simulink model "TruckBenchmark"  (R2023a)
settings: Solver=FixedStepAuto  StartTime=0.0  StopTime=sim_time  FixedStep=control.Ts  MaxStep=1  RelTol=1e-3  EnableMultiTasking=on
StartFcn:
  | tic
StopFcn:
  | simt=toc;
  | fprintf('Simulation time %.3f s\n',simt)
  | TruckBenchmark_Evaluation
values from neighbouring files (symbols this model uses):
  attack_duration = input('Enter the duration of each attack: ')    [RunMe.m]
  attack_freq = input('Enter the desired frequency of attack: ')    [RunMe.m]
  attack_time = input('Enter the time for attack: ')    [RunMe.m]
  attack_type = input('Select the type of Attack (1= Fuzzy, 2=spoofing, 3=Plateau, 4=Replay Attack, 5 = GAttack, 6= C-GAttack, 7= No Attack, 8 = Denial of Service):')    [RunMe.m]
  can_sample_time = 0.001    [runSim.m]
  clutch_pos = TruckBenchmark_Result.find('clutch_pos').Values    [TruckBenchmark_Evaluation.m]
  control =     [TruckBenchmark_Control.mat]
  cruise_profile = input('Select Cruise Profile (Step decrease = 1, Constant 80kph = 2): ')    [RunMe.m]
  curr_gear = TruckBenchmark_Result.find('curr_gear').Values    [TruckBenchmark_Evaluation.m]
  DoS = 0    [RunMe.m]
  gattack_data = interp1(original_time, data, desired_time, 'linear')    [RunMe.m]
  gattack_time = desired_time    [RunMe.m]
  k_slope = TruckBenchmark_Result.find('k_slope').Values    [TruckBenchmark_Evaluation.m]
  lambda = TruckBenchmark_Result.find('lambda').Values    [TruckBenchmark_Evaluation.m]
  model =     [TruckBenchmark_Data.mat]
  n_engine = TruckBenchmark_Result.find('n_engine').Values    [TruckBenchmark_Evaluation.m]
  road = scenario.road    [runSim.m]
  scenario =     [Sodertalje_Norrkoping_Scenario.mat]
  sim_time = input('Enter the total simulation time: ')    [RunMe.m]
  spoofed_value = input('Set the spoofing value:')    [RunMe.m]
  ts = struct('orig_30kph', ts_orig_30kph, 'gen_30kph', ts_gen_30kph, 'orig_40kph', ts_orig_40kph, 'gen_40kph', ts_gen_40kph, 'orig_50kph', ts_orig_50kph, 'gen_50kph', ts_gen_50kph, 'orig_60kph', ts_orig_60kph, 'gen_60kph', ts_gen_60kph,'orig_70kph', ts_orig_70kph, 'gen_70kph', ts_gen_70kph, 'orig_80kph', ts_orig_80kph, 'gen_80kph', ts_gen_80kph, 'orig_90kph', ts_orig_90kph, 'gen_90kph', ts_gen_90kph)    [data_to_mat.m]
  v_vehicle = 0    [RunMe.m]    (also in TruckBenchmark_Evaluation.m = TruckBenchmark_Result.find('v_vehicle').Values)
undefined symbols (not defined in the file or in its folder): canChannel, CCVS, DiscIntNeverNeededParam, dm_airInlet, EGF1, ESSI, ETC2, gcbh, IMT1, n_t, p_inletManifold, r_egr, VD, VDHR, x_distance
libraries: j1939protocollib x25, simulink x5, canlib x2, j1939tllib x2, canmsglib x1, vntj1939tllib x1, slpidlib x1
(part 4 of 4)

== system TruckBenchmark/Vehicle Model/ICE/Turbo/Turbine/eta_tm ==
  omega_t : Inport
  T_em : Inport  Port=2
  PI_t : Inport  Port=3
  BSR : Fcn  Expr=R_t*u[1]/sqrt(2*c_pe*u[2]*(1-u[3]^(1-1/gamma_e)))
  Fcn eta_t : Fcn  Expr=eta_tmmax-u[1]*(u[2]-BSR_opt)^2
  Mux1 : Mux  Inputs=2
  Mux4 : Mux  Inputs=3
  Saturation : Saturate  UpperLimit=2*BSR_opt  LowerLimit=0
  Saturation1 : Saturate  UpperLimit=1  LowerLimit=0.2
  c_m : Subsystem
  eta_tm : Outport  VectorParamsAs1DForOutWhenUnconnected=off
  tag scope: BSR=global
  wires:
  c_m/1(c_m) -> Mux1/1
  Saturation/1 -> [BSR], Mux1/2
  Mux1/1 -> Fcn eta_t/1
  Saturation1/1 -> eta_tm/1
  Fcn eta_t/1 -> Saturation1/1
  PI_t/1 -> Mux4/3
  T_em/1 -> Mux4/2
  omega_t/1 -> c_m/1(omega_t), Mux4/1
  BSR/1 -> Saturation/1
  Mux4/1 -> BSR/1

== system TruckBenchmark/Vehicle Model/ICE/Turbo/Compressor/DeltaT_c/eta_c ==
  W_c : Inport
  PI_c : Inport  Port=2
  Constant2 : Constant  Value=0.2
  Fcn eta_c : Fcn  Expr=eta_cmax-u
  Matrix Gain : Gain  Gain=Q_c  Multiplication=Matrix(K*u)  SaturateOnIntegerOverflow=on  OutDataTypeStr=Inherit: Same as input  ParamDataTypeStr=Inherit: Same as input
  MinMax2 : MinMax  Function=max  Inputs=2  InputSameDT=on  SaturateOnIntegerOverflow=on
  Mux6 : Mux  Inputs=2
  Product : Product  Multiplication=Matrix(*)  SaturateOnIntegerOverflow=on  OutDataTypeStr=Inherit: Same as first input
  chi1 : Fcn  Expr=u-w_copt
  chi2 : Fcn  Expr=u-pi_copt
  pi_c : Fcn  Expr=(u-1)^c_pi
  transp : Math  Operator=transpose  SignedPower=on
  eta_c : Outport  VectorParamsAs1DForOutWhenUnconnected=off
  wires:
  W_c/1 -> chi1/1
  MinMax2/1 -> eta_c/1
  PI_c/1 -> pi_c/1
  Constant2/1 -> MinMax2/2
  Fcn eta_c/1 -> MinMax2/1
  Product/1 -> Fcn eta_c/1
  Matrix Gain/1 -> Product/2
  transp/1 -> Product/1
  Mux6/1 -> transp/1, Matrix Gain/1
  chi2/1 -> Mux6/2
  chi1/1 -> Mux6/1
  pi_c/1 -> chi2/1

== system TruckBenchmark/Vehicle Model/ICE/Turbo/Compressor/Sub W_c/PHI_c ==
  PI_c : Inport
  T_bc : Inport  Port=2
  omega_t : Inport  Port=3
  Constant : Constant  Value=0
  Constant1 : Constant  Value=0
  Constant2 : Constant  Value=0
  Constant3 : Constant  Value=0.1
  MinMax{,1..3} (4 alike) : MinMax  Function=max  Inputs=2  InputSameDT=on  SaturateOnIntegerOverflow=on
  Mux1 : Mux  Inputs=2
  Mux2 : Mux  Inputs=2
  Mux5 : Mux  Inputs=3
  PSI_c : Fcn  Expr=2*c_pa*u[2]*(u[1]^(1-1/gamma_a)-1)/(R_c^2*u[3]^2)
  c_phi1 : Polyval  Coefs=c_wphiVec
  c_psi1 : Polyval  Coefs=c_wpsiVec
  fcn : Fcn  Expr=1-u[2]*(u[1]-c_psi2)^2
  fcn1 : Fcn  Expr=c_phi2+sqrt(u[1]/u[2])
  PHI_c : Outport  VectorParamsAs1DForOutWhenUnconnected=off
  wires:
  Constant3/1 -> MinMax3/2
  MinMax3/1 -> Mux2/2
  c_phi1/1 -> MinMax3/1
  MinMax2/1 -> PHI_c/1
  fcn1/1 -> MinMax2/2
  Constant2/1 -> MinMax2/1
  Mux2/1 -> fcn1/1
  MinMax/1 -> Mux2/1
  fcn/1 -> MinMax/2
  Constant/1 -> MinMax/1
  MinMax1/1 -> Mux1/2
  c_psi1/1 -> MinMax1/1
  Constant1/1 -> MinMax1/2
  Mux1/1 -> fcn/1
  PSI_c/1 -> Mux1/1
  omega_t/1 -> c_phi1/1, c_psi1/1, Mux5/3
  T_bc/1 -> Mux5/2
  PI_c/1 -> Mux5/1
  Mux5/1 -> PSI_c/1

== system TruckBenchmark/Vehicle Model/ICE/Turbo/Turbine/Sub W_t/f_vgt ==
  u_vgt : Inport
  Constant : Constant  Value=0
  Constant1 : Constant  Value=0
  Fcn f_vgt : Fcn  Expr=c_f2+c_f1*sqrt(u)
  Fcn1 : Fcn  Expr=1-((u-c_vgt2)/c_vgt1)^2
  MinMax : MinMax  Function=max  Inputs=2  InputSameDT=on  SaturateOnIntegerOverflow=on
  MinMax1 : MinMax  Function=max  Inputs=2  InputSameDT=on  SaturateOnIntegerOverflow=on
  f_vgt : Outport  VectorParamsAs1DForOutWhenUnconnected=off
  wires:
  MinMax1/1 -> f_vgt/1
  Fcn f_vgt/1 -> MinMax1/1
  Constant1/1 -> MinMax1/2
  MinMax/1 -> Fcn f_vgt/1
  Constant/1 -> MinMax/2
  Fcn1/1 -> MinMax/1
  u_vgt/1 -> Fcn1/1

== system TruckBenchmark/Vehicle Model/ICE/Turbo/Turbine/eta_tm/c_m ==
  omega_t : Inport
  Constant : Constant  Value=c_mVec(2)
  MinMax : MinMax  Function=max  Inputs=2  InputSameDT=on  SaturateOnIntegerOverflow=on
  Switch PSI : Switch  Threshold=w_tlin  InputSameDT=off
  c_m linear : Fcn  Expr=c_mlin*(u-c_mVec(2))/(w_tlin-c_mVec(2))
  c_m power : Fcn  Expr=c_mVec(1)*(u-c_mVec(2))^c_mVec(3)
  c_m : Outport  VectorParamsAs1DForOutWhenUnconnected=off
  wires:
  Switch PSI/1 -> c_m/1
  c_m linear/1 -> Switch PSI/3
  c_m power/1 -> Switch PSI/1
  omega_t/1 -> MinMax/2
  Constant/1 -> MinMax/1
  MinMax/1 -> c_m linear/1, Switch PSI/2, c_m power/1

== matlab function TruckBenchmark/Controller/Controller/cruise_set ==
  data: time input; cruise_set_speed output
function cruise_set_speed = switch_sig(time)
    % Define time constraint parameters
    %switch_time = 150; % Time to switch signals (in seconds)
    to = 100;
    % Initialize mux input
    cruise_set_speed = zeros(size(time));
    
    % Select signal 1 for the first part of the time vector
    if (time <= to )
        cruise_set_speed = 90;
    elseif (time > to && time<=to+50) 
        cruise_set_speed = 90;
    elseif (time > to+50 && time<=to+150) 
        cruise_set_speed = 80;
    elseif (time > to+150 && time<=to+250) 
        cruise_set_speed = 70;
    elseif (time > to+250 && time<=to+350) 
        cruise_set_speed = 60;
    elseif (time > to+350 && time<=to+450) 
        cruise_set_speed = 50;
    elseif (time > to+450 && time<=to+550) 
        cruise_set_speed = 40;
        %cruise_set_speed = 50;
    elseif (time > to+550) 
        cruise_set_speed = 30;
        %cruise_set_speed = 50;




    
    
end

== matlab function TruckBenchmark/Controller/CAN TX//RX/Attack_select ==
  data: GAttack input; output output; CGAttack input
function output = switch_sig(GAttack, CGAttack)
    % Define time constraint parameters
    switch_signal = attack_type; % Time to apply attack (no attack if at sim stop time)
    %switch_time = max(simTime); % Time to apply attack (Gattack)
    %switch_time = max(simTime); % Time to apply attack (CGattack)

    % Initialize mux input
    output = zeros(size(GAttack));
    
    % Select signal 1 for the first part of the time vector
    if (switch_signal == 1)
        output = GAttack;
    elseif (switch_signal == 2) 
        output = CGAttack;
    else
        output = 0;
    
    
end

== matlab function TruckBenchmark/Controller/CAN TX//RX/Attack Block/Attack_Block2 ==
  data: time input; mux_input output; attack_time input; attack_freq input; attack_duration input; sim_time input
function mux_input = switch_sig(time, attack_time, attack_freq, attack_duration, sim_time)
    % Initialize mux input as a vector of zeros with the same size as time
    mux_input = zeros(size(time));

    % Define the period between consecutive attacks
    attack_interval = (sim_time - attack_time) / (attack_freq);

    % Iterate through each time step
    for i = 1:length(time)
        % For each attack, determine if the time is within the attack period
        for j = 0:attack_freq-1
            current_attack_start = attack_time + j * attack_interval;
            current_attack_end = current_attack_start + attack_duration;
            
            % Check if the current time falls within the attack period
            if time(i) >= current_attack_start && time(i) <= current_attack_end
                mux_input(i) = 1;  % Set the signal to 1 during the attack
            end
        end
    end
end

== matlab function TruckBenchmark/Controller/Controller/P speed control ==
  data: v_ref input; v_speed input; u output; p_im input; curr_gear input; gear input; v_err output
function [u, v_err] = P(v_ref,v_speed,p_im,curr_gear,gear)
%#codegen


Kp      = 300;
v_err   = v_ref - v_speed;
u       = v_err * Kp;

% smoke limiter
K_smoke = 0.0012;
u_max=K_smoke*p_im;

% handle upshifts where the speed changes rapidly and the slowly sampled
% controller lags behind.
persistent last_gear second_last_gear

if isempty(last_gear)
  last_gear=4;
  second_last_gear=4;
end
if second_last_gear<curr_gear,
  u_max=u_max*.7;
end

second_last_gear=last_gear;
last_gear=curr_gear;
u=min(u,u_max);

== matlab function TruckBenchmark/Vehicle Model/Transmission Control Unit ==
  settings: updateMethod=DISCRETE
  data: gear_ref input; clutch output; gear_out output; time input
function [clutch,gear_out]  = TCU(gear_ref,time)
%#codegen
% Transmission control unit
persistent previous_gear incoming_gear last_state
persistent state t_start last_call
t_declutch=0.5;
t_speed_sync=1.0;
t_onclutch=0.5;


% run initialization
if isempty(state)
  % Initial state
  state=0;
  % Need to set varibles (some to dummy) so that codegen gets to know the size of the
  % persistent variables
  previous_gear=4;
  incoming_gear=4;
  t_start=0;
  previous_gear=gear_ref;
  last_call=time;
  last_state=state;
end
  
% Check if Simulink is restarting with smaller step reduction
if time < last_call,
  if state > 0,
    % disp(['Time reversed during gearchange']);
    if time - t_start < t_declutch,
      state=1;
    elseif time - t_start < t_declutch+t_speed_sync,
      state=2;
    elseif time - t_start < t_declutch+t_speed_sync+t_onclutch
      % backing state_machine
      state=3;
    else
      state=0;
    end
  end
end

last_call=time;
last_state=state;

% Run the state machine
switch state,
  case 0, % 'normal'
    if (gear_ref~=previous_gear)
      t_start=time;
      incoming_gear=gear_ref;
      state=1;
    end
    clutch=1;
    gear_out=previous_gear;
  case 1, % 'ramp_down',
    if ((time-t_start)>t_declutch)
      state=2;
      clutch=0;
    else
      clutch=1-(time-t_start)/t_declutch;
    end    
    gear_out=previous_gear;
  case 2, % 'change_gear',
    if (time>(t_start+t_declutch+t_speed_sync))
      state=3; % 'ramp_up';
      clutch=(time-(t_start+t_declutch+t_speed_sync))/t_onclutch;
    else
      clutch=0;
    end
    gear_out=incoming_gear;
  case 3, % 'ramp_up',
    if (time>(t_start+t_declutch+t_speed_sync+t_onclutch))
      state=0; %'normal';
      clutch=1;
    else
      clutch=(time-(t_start+t_declutch+t_speed_sync))/t_onclutch;
    end
    gear_out=incoming_gear;
    previous_gear=incoming_gear;
  otherwise
    error('Unknown state');
end

== matlab function TruckBenchmark/Vehicle Model/Fuel consumption dm^3//(100km) ==
  data: m_fuelTot input; x_distance input; fuelConsumption output
function fuelConsumption = fcn(m_fuelTot,x_distance)
%#codegen
rho_fuel = 0.8;                               % kg/m^2
if x_distance > 1000
    fuelConsumption = m_fuelTot / (rho_fuel * x_distance / 100000 );   % dm^3/(100km)
else
    fuelConsumption = nan;
end

== matlab function TruckBenchmark/Controller/Controller/PI speed control1 ==
  data: k_slopeVector input; k_slope output; x_distanceVector input; currentPos input
function k_slope = slope(k_slopeVector ,  x_distanceVector, currentPos)
%#codegen

% This function is not implemented.
k_slope      = 0;

== matlab function TruckBenchmark/Controller/Controller/Gear control ==
  data: n_ice input; gear_ref output; curr_gear input; clutch input
function gear_ref  = gearbox_control(n_ice, curr_gear, clutch)
%#codegen

% Define persistant variables
persistent curr_gear_ref

% initialize persistant variable
if isempty(curr_gear_ref)
    curr_gear_ref=4;
end

n_gearUpshift = 1250;
n_gearDoubleUpshift = 1800;
n_gearDownshift = 900;
gearMax   = 14;
gearMin   = 4;

if curr_gear_ref~=curr_gear || clutch~=1; %Gear in progress - keep current gear reference
    gear_ref = curr_gear_ref;     
elseif n_ice > n_gearUpshift && curr_gear < gearMax %Shift upp  
    if n_ice > n_gearDoubleUpshift && curr_gear < gearMax-1 %Shift up two gears
        gear_ref = curr_gear + 2;
    else % Shift up one gear
        gear_ref = curr_gear + 1;
    end 
elseif n_ice < n_gearDownshift && curr_gear > gearMin %Shift down
    gear_ref = curr_gear - 1;
else %No shift - keep current gear
    gear_ref = curr_gear;
end

gear_ref = min(max(gear_ref,gearMin),gearMax); %Should not be necissairy

curr_gear_ref=gear_ref;

== matlab function TruckBenchmark/Controller/Controller/PI speed control ==
  data: v_ref input; v_speed input; u output; p_im input; curr_gear input; gear input; v_err output; u_int input; u_diff input
function [u, v_err] = PI(v_ref,v_speed,p_im,curr_gear,gear, u_int, u_diff)
%#codegen
persistent last_v_err last_t

Kp      = 400;
Ki      = 0.05; % Increase the integration gain
Kd = 1;
v_err   = v_ref - v_speed;

% Integrate the error
if isempty(last_v_err)
    last_v_err = v_err;
    last_t = 0;
end
delta_t = 0.01; % Assuming a sampling time of 0.01 seconds
%u_int = (v_err + last_v_err) * delta_t / 2; % Trapezoidal integration
%u_int_max = 100; % Maximum integral component
%u_int = max(min(u_int, u_int_max), -u_int_max); % Limit the integral component
last_v_err = v_err;

%u = Kp * v_err + Ki * u_int + Kd * u_diff;
u = Kp * v_err + Ki * u_int;

% smoke limiter
K_smoke = 0.0012;
u_max=K_smoke*p_im;

% handle upshifts where the speed changes rapidly and the slowly sampled
% controller lags behind.
persistent last_gear second_last_gear

if isempty(last_gear)
  last_gear=4;
  second_last_gear=4;
end
if second_last_gear<curr_gear,
  u_max=u_max*.7;
end

second_last_gear=last_gear;
last_gear=curr_gear;
u=min(u,u_max);

== matlab function TruckBenchmark/Controller/CAN TX//RX/ Periodic Trigger1/Timer/MATLAB Function ==
  data: y output double
function y = fcn
%#codegen
persistent temp;
coder.extrinsic('tic')
if isempty(temp)
    tic;
    temp = 0;
end
coder.extrinsic('toc')
temp = toc;
y = temp;

== matlab function TruckBenchmark/Controller/CAN TX//RX/Attack_Block2 ==
  data: output output; cruise_speed input
function output = select_profile(cruise_speed)
    %fieldnames(data);
    
    data = load('attack_vehicle_velocity_RCGAN.mat');
    % Initialize output
    selectedField = '';
    %cruise_speed = ones(size(data.gen_30kph);
    % Selection logic based on cruise speed
    % Define speed thresholds and corresponding field names
    if cruise_speed <= 30
        selectedField = 'gen_30kph'; % Replace with actual field name
    elseif cruise_speed > 30 && cruise_speed <= 40
        selectedField = 'gen_40kph'; % Replace with actual field name
    elseif cruise_speed > 40 && cruise_speed <= 50
        selectedField = 'gen_50kph'; % Replace with actual field name
    elseif cruise_speed > 50 && cruise_speed <= 60
        selectedField = 'gen_60kph'; % Replace with actual field name
    elseif cruise_speed > 60 && cruise_speed <= 70
        selectedField = 'gen_70kph'; % Replace with actual field name
    elseif cruise_speed > 70 && cruise_speed <= 80
        selectedField = 'gen_80kph'; % Replace with actual field name
    elseif cruise_speed > 80 && cruise_speed <= 90
        selectedField = 'gen_90kph'; % Replace with actual field name
    else
        error('Cruise speed out of supported range');
    end
    
    % % Ensure that the selected field exists
    % if isfield(data.ts, selectedField)
    %     output = data.ts.(selectedField);
    % else
    %     error('Selected field does not exist in the data structure.');
    % end

    % Extract the selected time series data
    output = data.ts.(selectedField); 
end

== matlab function TruckBenchmark/Controller/CAN TX//RX/Attack Block/Attack_Block1 ==
  data: time input; mux_input output; attack_time input
function mux_input = switch_sig(time, attack_time)
    % Define time constraint parameters
    switch_time = attack_time; % Time to apply attack (no attack if at sim stop time)
    %switch_time = max(simTime); % Time to apply attack (Gattack)
    %switch_time = max(simTime); % Time to apply attack (CGattack)

    % Initialize mux input
    mux_input = zeros(size(time));
    
    % Select signal 1 for the first part of the time vector
    if (time >= switch_time)
        mux_input = 1;
    else 
        mux_input = 0;
    
    
end
